simulink model "controllableSource"  (R2023a)
settings: Solver=ode3  StartTime=0.0  StopTime=2  FixedStep=HWSampleTime  RelTol=1e-3
undefined symbols (not defined in the file or in its folder): DiscIntNeverNeededParam, VScourceData
libraries: nesl_utility x4, ee_lib x3, fl_lib x2, eeTransforms x1
settings Model: Creator=e2n051  LastModifiedBy=e2n051

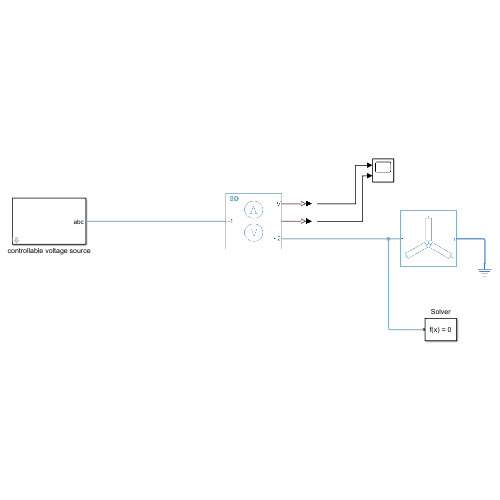
[thumbnail: Simulink's stored preview of the top-level diagram]
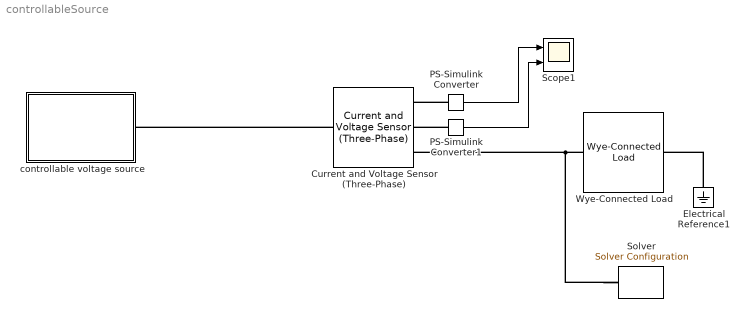
== system controllableSource ==
  Current and Voltage Sensor (Three-Phase) : ee_lib/Sensors & Transducers/Current and Voltage Sensor (Three-Phase)  vMeasurementType=ee.enum.vmeasurement.lg  outputUnit=ee.enum.unit.si  SRated=100e6 A*V  VRated=24e3 V  I_specify=off  I_priority=None  I=[0, 0, 0] A  I_nominal_specify=off  I_nominal_unit=A  I_nominal_value=1  V_specify=off  V_priority=None  V=[0, 0, 0] V  V_nominal_specify=off  V_nominal_unit=V  V_nominal_value=1
      settings: InternalSimscapePortConfiguration="{\"Bottom\":[],\"Left\":[{\"id\":\"N1\",\"label\":\"~1\",\"type\":\"foundation.electrical.three_phase\"}],\"Right\":[{\"id\":\"V_output\",\"label\":\"V\",\"type\":\"output\"},{\"id\":\"I_output\",\"label\":\"I\",\"type\":\"output\"},{\"id\":\"N2\",\"label\":\"~2\",\"type\":\"foundation.electrical.three_phase\"}],\"Top\":[]}"
  Electrical Reference1 : fl_lib/Electrical/Electrical Elements/Electrical Reference
  PS-Simulink Converter : nesl_utility/PS-Simulink Converter  PhysicalDomain=network_engine_domain  SubClassName=ps_output  LeftPortType=input  RightPortType=output  PseudoPeriodic=off  Frequencies=[]  VectorFormat=inherit  Unit=inherit  AffineConversion=off
  PS-Simulink Converter1 : nesl_utility/PS-Simulink Converter  PhysicalDomain=network_engine_domain  SubClassName=ps_output  LeftPortType=input  RightPortType=output  PseudoPeriodic=off  Frequencies=[]  VectorFormat=inherit  Unit=inherit  AffineConversion=off
  Scope1 : Scope  NumInputPorts=2
  Solver : nesl_utility/Solver Configuration  PhysicalDomain=network_engine_domain  SubClassName=solver  LeftPortType=input  RightPortType=generic  Tones=[]  Harmonics=[]  SimulateNoise=off  Profile=off  UseLocalSampling=off  EnableSwitchedLinearOptims=on  FrequencyDomain=off  UseCCode=off  RelTol=0.001  AbsTol=1e-06  MinStep=1e-09  ToWorkspace=off  RevertToSquareIcSolve=off  NumHomotopyIterations=100  PhasorMode=off  PhasorModeNumHarmonics=1  ConsistencySolver=NEWTON_FTOL  IndexReductionMethod=DerivativeReplacement  DoDC=off  ResidualTolerance=1e-2  ConsistencyTolSource=GLOBAL  ConsistencyAbsTol=0.001  ConsistencyRelTol=0.001  ConsistencyTolFactor=0.001  UseLocalSolver=on  LocalSolverChoice=NE_BACKWARD_EULER_ADVANCER  ResolveIndetEquations=on  FunctionEvalNumThread=1  LocalSolverSampleTime=HWSampleTime  DoFixedCost=off  MaxNonlinIter=3  MaxModeIter=2  ComputeImpulses=off  ImpulseIterations=2  LinearAlgebra=Sparse  LinearAlgebraNumThread=0  EquationFormulation=NE_TIME_EF  DelaysMemoryBudget=1024  AutomaticFiltering=on  FilteringTimeConstant=0.001  PartitionStorageMethod=AS_NEEDED  PartitionMemoryBudget=1024  PartitionMethod=FAST
  Wye-Connected Load : ee_lib/Passive/RLC Assemblies/Wye-Connected Load  parameterization=ee.enum.rlc.parameterization.ratedpower  component_structure=ee.enum.rlc.structure.R  component_structure_PQ=ee.enum.rlc.structure.R  R=1 Ohm  L=1e-3 H  C=1e-6 F  VRated=230 V  FRated=60 Hz  P=1e3 W  Qpos=1e2 A*V  Qneg=-1e2 A*V  R_parasitic=0 Ohm  G_parasitic=0 1/Ohm  R_parasitic_PQ=0 Ohm  G_parasitic_PQ=0 1/Ohm  Vmag0=24e3 V  Vang0=0 deg  Freq0=60 Hz  IL_specify=off  IL_priority=High  IL=[0, 0, 0] A  IL_nominal_specify=off  IL_nominal_unit=A  IL_nominal_value=1  VC_specify=off  VC_priority=High  VC=[0, 0, 0] V  VC_nominal_specify=off  VC_nominal_unit=V  VC_nominal_value=1
  controllable voltage source : Subsystem  mask{Vscource_data=VScourceData}
      mask prompts: Vscource_data "all_variables"
  wires:
  PS-Simulink Converter/1 -> Scope1/1
  PS-Simulink Converter1/1 -> Scope1/2
  connections:
  PS-Simulink Converter/LConn1 -- Current and Voltage Sensor (Three-Phase)/RConn1
  Wye-Connected Load/LConn1 -- Solver/RConn1 -- Current and Voltage Sensor (Three-Phase)/RConn3
  PS-Simulink Converter1/LConn1 -- Current and Voltage Sensor (Three-Phase)/RConn2
  Electrical Reference1/LConn1 -- Wye-Connected Load/RConn1
  Current and Voltage Sensor (Three-Phase)/LConn1 -- controllable voltage source/RConn1

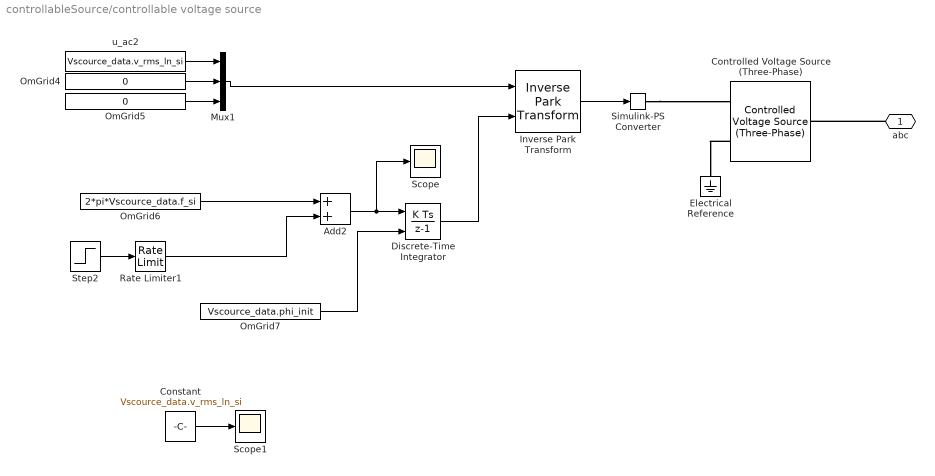
== system controllableSource/controllable voltage source ==
  Add2 : Sum
  Constant : Constant  Value=Vscource_data.v_rms_ln_si
  Controlled Voltage Source (Three-Phase) : ee_lib/Sources/Controlled Voltage Source (Three-Phase)  input_option=ee.enum.inputType.instantaneous  FRated=60 Hz
      settings: InternalSimscapePortConfiguration="{\"Bottom\":[],\"Left\":[{\"id\":\"S\",\"label\":\"S\",\"type\":\"input\"},{\"id\":\"n\",\"label\":\"n\",\"type\":\"foundation.electrical.electrical\"}],\"Right\":[{\"id\":\"N\",\"label\":\"~\",\"type\":\"foundation.electrical.three_phase\"}],\"Top\":[]}"
  Discrete-Time Integrator : DiscreteIntegrator  InitialConditionSource=external  SampleTime=-1  ICPrevOutput=DiscIntNeverNeededParam  ICPrevScaledInput=DiscIntNeverNeededParam
  Electrical Reference : fl_lib/Electrical/Electrical Elements/Electrical Reference
  Inverse Park Transform : eeTransforms/Inverse Park Transform  AxisAlignment=Q-axis  PowerInvariant=off
      settings: LibrarySourceBlock=|
      | ee_sl_lib/Mathematical
      | Transforms/Inverse
      | Park Transform
  Mux1 : Mux  Inputs=3
  OmGrid4 : Constant  Value=0
  OmGrid5 : Constant  Value=0
  OmGrid6 : Constant  Value=2*pi*Vscource_data.f_si
  OmGrid7 : Constant  Value=Vscource_data.phi_init
  Rate Limiter1 : RateLimiter  RisingSlewLimit=2*pi*Vscource_data.rocof_des_si  FallingSlewLimit=-2*pi*Vscource_data.rocof_des_si  SampleTimeMode=inherited
  Scope : Scope
  Scope1 : Scope
  Simulink-PS Converter : nesl_utility/Simulink-PS Converter  PhysicalDomain=network_engine_domain  SubClassName=ps_input  LeftPortType=input  RightPortType=output  PseudoPeriodic=off  Frequencies=[]  NoiseDistribution=none  NoiseParameters=[]  Unit=1  AffineConversion=off  FilteringAndDerivatives=provide  SimscapeFilterOrder=1  InputFilterTimeConstant=0.001  UdotUserProvided=0
  Step2 : Step  Time=Vscource_data.t_rocof  After=2*pi*Vscource_data.max_f_dev_si  SampleTime=0
  u_ac2 : Constant  Value=Vscource_data.v_rms_ln_si
  abc : PMIOPort  Side=Right
  wires:
  OmGrid5/1 -> Mux1/3
  Mux1/1 -> Inverse Park Transform/1
  u_ac2/1 -> Mux1/1
  OmGrid4/1 -> Mux1/2
  Inverse Park Transform/1 -> Simulink-PS Converter/1
  Discrete-Time Integrator/1 -> Inverse Park Transform/2
  OmGrid7/1 -> Discrete-Time Integrator/2
  Step2/1 -> Rate Limiter1/1
  OmGrid6/1 -> Add2/1
  Add2/1 -> Scope/1, Discrete-Time Integrator/1
  Rate Limiter1/1 -> Add2/2
  Constant/1 -> Scope1/1
  connections:
  Simulink-PS Converter/RConn1 -- Controlled Voltage Source (Three-Phase)/LConn1
  Controlled Voltage Source (Three-Phase)/LConn2 -- Electrical Reference/LConn1
  abc/RConn1 -- Controlled Voltage Source (Three-Phase)/RConn1
